simulink model "Boiler_System_Model"  (R2026a)
settings: Solver=ode15s  StopTime=1000
undefined symbols (not defined in the file): Flow_Min_LPM, P_Boost_W, P_Internal_W, Solar_Gain_Coeff, T_Ambient_C, T_Initial_C, T_Max_Cutoff_C, T_solar, T_standby, T_target_logic, T_Water_Inlet_C, UA_Losses, Water_Mass_kg
libraries: fl_lib x10, nesl_utility x7, simulink x3
settings Model: Creator=eladmual  LastModifiedBy=User
settings SolverCC: ZeroCrossAlgorithm=Adaptive
settings DebuggingCC: IgnoredZcDiagnostic=none
settings SimscapeCC: SimscapeNominalValues="[{\"value\":\"1\",\"unit\":\"A\"},{\"value\":\"1\",\"unit\":\"bar\"},{\"value\":\"1\",\"unit\":\"cm^2\"},{\"value\":\"1\",\"unit\":\"cm^3/s\"},{\"value\":\"1\",\"unit\":\"kJ/kg\"},{\"value\":\"1\",\"unit\":\"kW\"},{\"value\":\"1\",\"unit\":\"l\"},{\"value\":\"1\",\"unit\":\"N\"},{\"value\":\"1\",\"unit\":\"N*m\"},{\"value\":\"1\",\"unit\":\"V\"}]"  SimscapeLogType=none  SimscapeLogDataHistory=5000.0

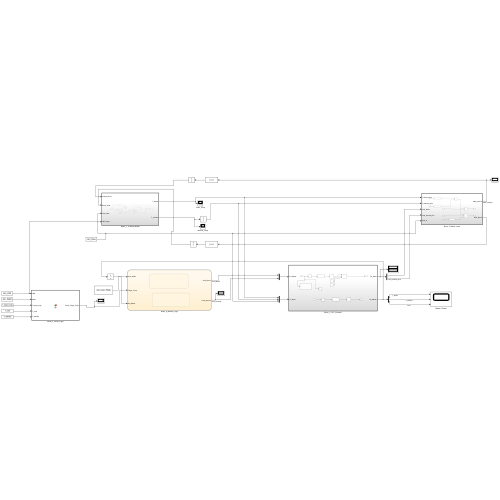
[thumbnail: Simulink's stored preview of the top-level diagram]
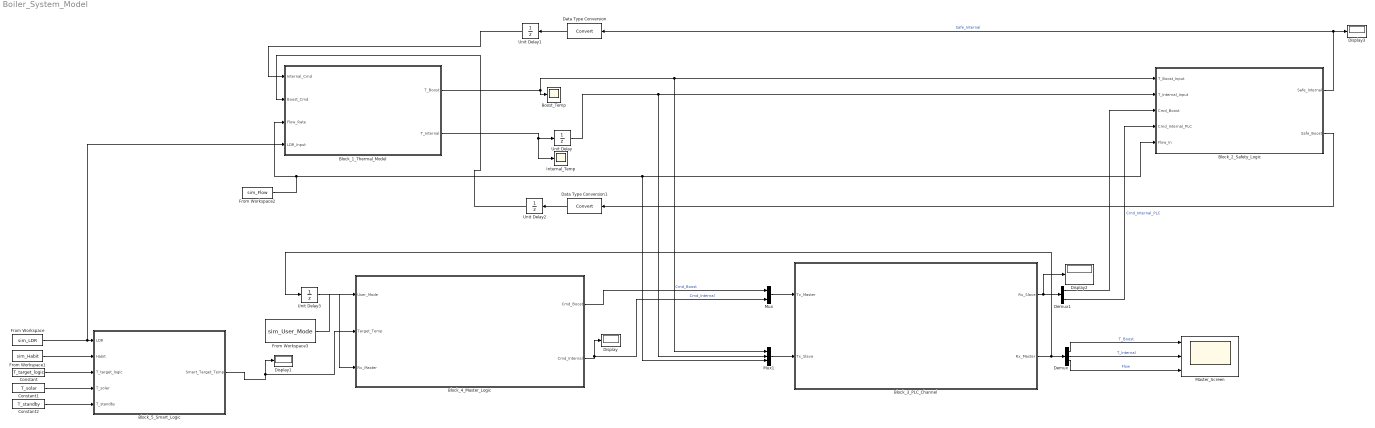
== system Boiler_System_Model ==
  Block_1_Thermal_Model : Subsystem  TreatAsAtomicUnit=on
  Block_2_Safety_Logic : Subsystem  TreatAsAtomicUnit=on
  Block_3_PLC_Channel : Subsystem  TreatAsAtomicUnit=on
  Block_4_Master_Logic : Stateflow chart  TreatAsAtomicUnit=on
  Block_5_Smart_Logic : MATLAB Function  TreatAsAtomicUnit=on
  Boost_Temp : Scope
      settings: ActiveDisplayYMinimum=8.9226285508408516  ActiveDisplayYMaximum=188.34662587796339
  Constant : Constant  Value=T_target_logic
  Constant1 : Constant  Value=T_solar
  Constant2 : Constant  Value=T_standby
  Data Type Conversion : DataTypeConversion  SaturateOnIntegerOverflow=off  RndMeth=Floor
  Data Type Conversion1 : DataTypeConversion  SaturateOnIntegerOverflow=off  RndMeth=Floor
  Demux : Demux  Outputs=3
  Demux1 : Demux  Outputs=2
  Display{,1..3} (4 alike) : Display
  From Workspace : FromWorkspace  VariableName=sim_LDR
  From Workspace1 : FromWorkspace  VariableName=sim_Habit
  From Workspace2 : FromWorkspace  VariableName=sim_Flow
  From Workspace3 : FromWorkspace  VariableName=sim_User_Mode
  Internal_Temp : Scope
      settings: ActiveDisplayYMinimum=25.95597381713398  ActiveDisplayYMaximum=34.896235645794405
  Master_Screen : Scope  NumInputPorts=3
      settings: ActiveDisplayYMinimum=0  ActiveDisplayYMaximum=70  DataLoggingVariableName=ScopeData2
  Mux : Mux  Inputs=2
  Mux1 : Mux  Inputs=3
  Unit Delay : UnitDelay  InitialCondition=20  SampleTime=-1
  Unit Delay1 : UnitDelay  InitialCondition=20  SampleTime=0.1
  Unit Delay2 : UnitDelay  InitialCondition=20  SampleTime=0.1
  Unit Delay3 : UnitDelay  SampleTime=-1
  wires:
  Block_1_Thermal_Model/2(T_Internal) -> Unit Delay/1, Internal_Temp/1
  From Workspace2/1 -> Mux1/3, Block_2_Safety_Logic/5(Flow_In), Block_1_Thermal_Model/3(Flow_Rate)
  Block_2_Safety_Logic/1(Safe_Internal) -> Data Type Conversion/1, Display3/1  "Safe_Internal"
  Block_2_Safety_Logic/2(Safe_Boost) -> Data Type Conversion1/1
  Data Type Conversion1/1 -> Unit Delay2/1
  Data Type Conversion/1 -> Unit Delay1/1
  Unit Delay/1 -> Mux1/2, Block_2_Safety_Logic/2(T_Internal_Input)
  Block_1_Thermal_Model/1(T_Boost) -> Boost_Temp/1, Mux1/1, Block_2_Safety_Logic/1(T_Boost_Input)
  Unit Delay1/1 -> Block_1_Thermal_Model/1(Internal_Cmd)
  Unit Delay2/1 -> Block_1_Thermal_Model/2(Boost_Cmd)
  Mux/1 -> Block_3_PLC_Channel/1(Tx_Master)
  Block_3_PLC_Channel/1(Rx_Slave) -> Display2/1, Demux1/1
  Mux1/1 -> Block_3_PLC_Channel/2(Tx_Slave)
  Demux/1 -> Master_Screen/1  "T_Boost"
  Demux/2 -> Master_Screen/2  "T_Internal"
  Demux/3 -> Master_Screen/3  "Flow"
  From Workspace3/1 -> Block_4_Master_Logic/1(User_Mode)
  Block_3_PLC_Channel/2(Rx_Master) -> Unit Delay3/1, Demux/1
  Block_4_Master_Logic/1(Cmd_Boost) -> Mux/1  "Cmd_Boost"
  Block_4_Master_Logic/2(Cmd_Internal) -> Display/1, Mux/2  "Cmd_Internal"
  Unit Delay3/1 -> Block_4_Master_Logic/3(Rx_Master)
  From Workspace/1 -> Block_5_Smart_Logic/1(LDR), Block_1_Thermal_Model/4(LDR_Input)
  From Workspace1/1 -> Block_5_Smart_Logic/2(Habit)
  Block_5_Smart_Logic/1(Smart_Target_Temp) -> Display1/1, Block_4_Master_Logic/2(Target_Temp)
  Demux1/1 -> Block_2_Safety_Logic/3(Cmd_Boost)
  Demux1/2 -> Block_2_Safety_Logic/4(Cmd_Internal_PLC)  "Cmd_Internal_PLC"
  Constant/1 -> Block_5_Smart_Logic/3(T_target_logic)
  Constant1/1 -> Block_5_Smart_Logic/4(T_solar)
  Constant2/1 -> Block_5_Smart_Logic/5(T_standby)

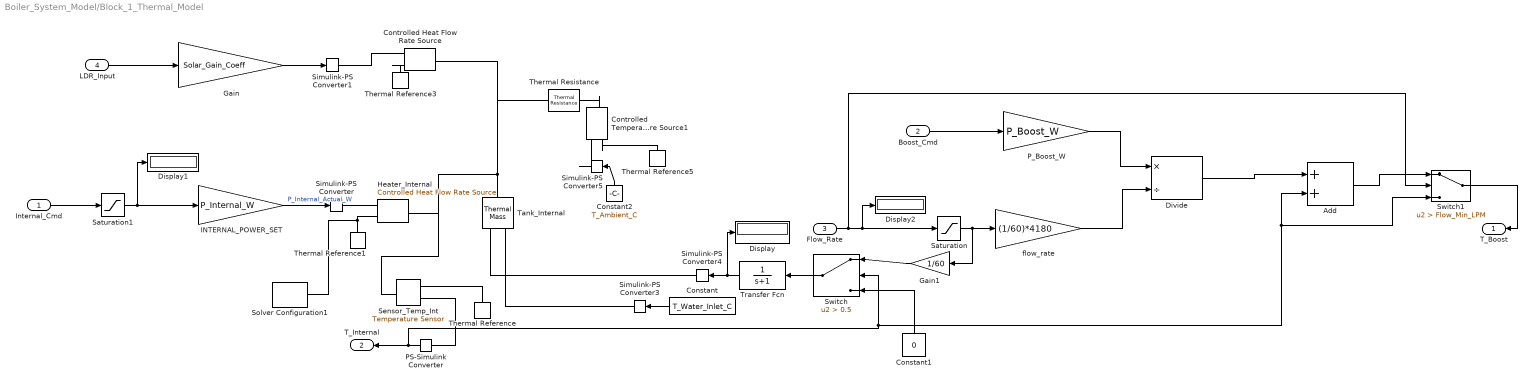
== system Boiler_System_Model/Block_1_Thermal_Model ==
  Internal_Cmd : Inport
  Boost_Cmd : Inport  Port=2
  Flow_Rate : Inport  Port=3
  LDR_Input : Inport  Port=4
  Add : Sum
  Constant : Constant  Value=T_Water_Inlet_C
  Constant1 : Constant  Value=0
  Constant2 : Constant  Value=T_Ambient_C
  Controlled Temperature Source1 : fl_lib/Thermal/Thermal Sources/Controlled Temperature Source
  Controlled Heat Flow Rate Source : fl_lib/Thermal/Thermal Sources/Controlled Heat Flow Rate Source
  Display : Display
  Display1 : Display
  Display2 : Display
  Divide : Product  Inputs=*/
  Gain : Gain  Gain=Solar_Gain_Coeff
  Gain1 : Gain  Gain=1/60
  Heater_Internal : fl_lib/Thermal/Thermal Sources/Controlled Heat Flow Rate Source
  INTERNAL_POWER_SET : Gain  Gain=P_Internal_W
  PS-Simulink Converter : nesl_utility/PS-Simulink Converter  PhysicalDomain=network_engine_domain  SubClassName=ps_output  LeftPortType=input  RightPortType=output  PseudoPeriodic=off  Frequencies=[]  VectorFormat=inherit  Unit=degC  AffineConversion=on
  P_Boost_W : Gain  Gain=P_Boost_W
  Saturation : Saturate  UpperLimit=inf  LowerLimit=0.001
  Saturation1 : Saturate  UpperLimit=1  LowerLimit=0
  Sensor_Temp_Int : fl_lib/Thermal/Thermal Sensors/Temperature Sensor  temperature_measure=foundation.enum.MeasurementReference.difference
  Simulink-PS Converter : nesl_utility/Simulink-PS Converter  PhysicalDomain=network_engine_domain  SubClassName=ps_input  LeftPortType=input  RightPortType=output  PseudoPeriodic=off  Frequencies=[]  NoiseDistribution=none  NoiseParameters=[]  Unit=W  AffineConversion=on  FilteringAndDerivatives=provide  SimscapeFilterOrder=1  InputFilterTimeConstant=0.001  UdotUserProvided=0
  Simulink-PS Converter1 : nesl_utility/Simulink-PS Converter  PhysicalDomain=network_engine_domain  SubClassName=ps_input  LeftPortType=input  RightPortType=output  PseudoPeriodic=off  Frequencies=[]  NoiseDistribution=none  NoiseParameters=[]  Unit=1  AffineConversion=off  FilteringAndDerivatives=provide  SimscapeFilterOrder=1  InputFilterTimeConstant=0.001  UdotUserProvided=0
  Simulink-PS Converter3 : nesl_utility/Simulink-PS Converter  PhysicalDomain=network_engine_domain  SubClassName=ps_input  LeftPortType=input  RightPortType=output  PseudoPeriodic=off  Frequencies=[]  NoiseDistribution=none  NoiseParameters=[]  Unit=1  AffineConversion=off  FilteringAndDerivatives=provide  SimscapeFilterOrder=1  InputFilterTimeConstant=0.001  UdotUserProvided=0
  Simulink-PS Converter4 : nesl_utility/Simulink-PS Converter  PhysicalDomain=network_engine_domain  SubClassName=ps_input  LeftPortType=input  RightPortType=output  PseudoPeriodic=off  Frequencies=[]  NoiseDistribution=none  NoiseParameters=[]  Unit=1  AffineConversion=off  FilteringAndDerivatives=provide  SimscapeFilterOrder=1  InputFilterTimeConstant=0.001  UdotUserProvided=0
  Simulink-PS Converter5 : nesl_utility/Simulink-PS Converter  PhysicalDomain=network_engine_domain  SubClassName=ps_input  LeftPortType=input  RightPortType=output  PseudoPeriodic=off  Frequencies=[]  NoiseDistribution=none  NoiseParameters=[]  Unit=degC  AffineConversion=on  FilteringAndDerivatives=provide  SimscapeFilterOrder=1  InputFilterTimeConstant=0.001  UdotUserProvided=0
  Solver Configuration1 : nesl_utility/Solver Configuration  PhysicalDomain=network_engine_domain  SubClassName=solver  LeftPortType=input  RightPortType=generic  Tones=[]  Harmonics=[]  SimulateNoise=off  Profile=off  UseLocalSampling=off  EnableSwitchedLinearOptims=on  FrequencyDomain=off  UseCCode=off  RelTol=0.001  AbsTol=0.001  MinStep=1e-09  ToWorkspace=off  RevertToSquareIcSolve=off  NumHomotopyIterations=100  PhasorMode=off  PhasorModeNumHarmonics=1  ConsistencySolver=NEWTON_XTOL_AFTER_FTOL  CanonicalOrdering=UNORDERED  OptimizeIntermediates=UNOPTIMIZED  IndexReductionMethod=DerivativeReplacement  DoDC=off  ResidualTolerance=1e-09  ConsistencyTolSource=GLOBAL  ConsistencyAbsTol=0.001  ConsistencyRelTol=0.001  ConsistencyTolFactor=0.001  UseLocalSolver=off  LocalSolverChoice=NE_BACKWARD_EULER_ADVANCER  ResolveIndetEquations=on  FunctionEvalNumThread=1  LocalSolverSampleTime=0.001  DoFixedCost=off  MaxNonlinIter=3  MaxModeIter=2  ComputeImpulses=off  ImpulseIterations=2  LinearAlgebra=auto  LinearAlgebraNumThread=0  EquationFormulation=NE_TIME_EF  DelaysMemoryBudget=1024  AutomaticFiltering=on  FilteringTimeConstant=0.001  PartitionStorageMethod=AS_NEEDED  PartitionMemoryBudget=1024  PartitionMethod=ROBUST  MultibodyUseLocalSolver=off  MultibodyLocalSolverChoice=ODE1  MultibodyLocalSolverSampleTime=0.001
  Switch : Switch  Criteria=u2 > Threshold  Threshold=0.5  ZeroCross=off  SaturateOnIntegerOverflow=off  InputSameDT=off
  Switch1 : Switch  Criteria=u2 > Threshold  Threshold=Flow_Min_LPM  SaturateOnIntegerOverflow=off  InputSameDT=off
  Tank_Internal : fl_lib/Thermal/Thermal Elements/Thermal Mass  mass_type=foundation.enum.constant_variable.variable  mass=Water_Mass_kg kg  sp_heat=4184 J/(K*kg)  mass_min=1 kg  num_ports=foundation.enum.numPorts2.one  m_specify=on  m_priority=High  m=Water_Mass_kg kg  m_nominal_specify=off  m_nominal_value=1  m_nominal_unit=kg  T_specify=on  T_priority=High  T=T_Initial_C degC  T_nominal_specify=off  T_nominal_value=1  T_nominal_unit=K  Q_specify=off  Q_priority=None  Q=0 W  Q_nominal_specify=off  Q_nominal_value=1  Q_nominal_unit=W
  Thermal Reference{,1,3,5} (4 alike) : fl_lib/Thermal/Thermal Elements/Thermal Reference
  Thermal Resistance : fl_lib/Thermal/Thermal Elements/Thermal Resistance  resistance=1/UA_Losses K/W  T_specify=off  T_priority=None  T=0 K  T_nominal_specify=off  T_nominal_value=1  T_nominal_unit=K  Q_specify=off  Q_priority=None  Q=0 W  Q_nominal_specify=off  Q_nominal_value=1  Q_nominal_unit=W
  Transfer Fcn : TransferFcn  Denominator=[1 1]
  flow_rate : Gain  Gain=(1/60)*4180
  T_Boost : Outport  Unit=degC
  T_Internal : Outport  Port=2  Unit=°C
  wires:
  Boost_Cmd/1 -> P_Boost_W/1
  INTERNAL_POWER_SET/1 -> Simulink-PS Converter/1  "P_Internal_Actual_W"
  P_Boost_W/1 -> Divide/1
  flow_rate/1 -> Divide/2
  PS-Simulink Converter/1 -> Switch/2, Switch1/3, Add/2, T_Internal/1
  Divide/1 -> Add/1
  LDR_Input/1 -> Gain/1
  Flow_Rate/1 -> Switch1/2, Display2/1, Saturation/1
  Saturation/1 -> Gain1/1, flow_rate/1
  Gain/1 -> Simulink-PS Converter1/1
  Constant/1 -> Simulink-PS Converter3/1
  Gain1/1 -> Switch/1
  Constant1/1 -> Switch/3
  Switch/1 -> Transfer Fcn/1
  Transfer Fcn/1 -> Display/1, Simulink-PS Converter4/1
  Add/1 -> Switch1/1
  Constant2/1 -> Simulink-PS Converter5/1
  Internal_Cmd/1 -> Saturation1/1
  Saturation1/1 -> INTERNAL_POWER_SET/1, Display1/1
  Switch1/1 -> T_Boost/1
  connections:
  Sensor_Temp_Int/LConn1 -- Heater_Internal/LConn1 -- Thermal Resistance/LConn1 -- Controlled Heat Flow Rate Source/LConn1 -- Tank_Internal/LConn1
  Simulink-PS Converter/RConn1 -- Heater_Internal/RConn1
  PS-Simulink Converter/LConn1 -- Sensor_Temp_Int/RConn2
  Heater_Internal/RConn2 -- Solver Configuration1/RConn1 -- Thermal Reference1/LConn1
  Sensor_Temp_Int/RConn1 -- Thermal Reference/LConn1
  Controlled Heat Flow Rate Source/RConn1 -- Simulink-PS Converter1/RConn1
  Controlled Heat Flow Rate Source/RConn2 -- Thermal Reference3/LConn1
  Tank_Internal/RConn2 -- Simulink-PS Converter3/RConn1
  Tank_Internal/RConn1 -- Simulink-PS Converter4/RConn1
  Controlled Temperature Source1/LConn1 -- Thermal Resistance/RConn1
  Simulink-PS Converter5/RConn1 -- Controlled Temperature Source1/RConn1
  Controlled Temperature Source1/RConn2 -- Thermal Reference5/LConn1

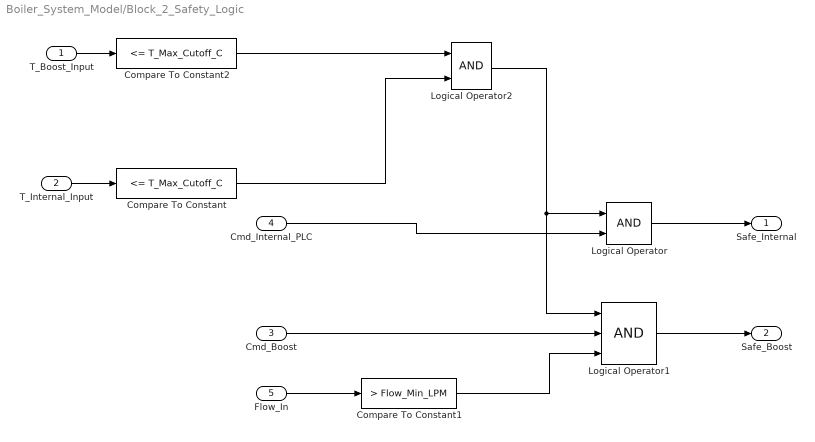
== system Boiler_System_Model/Block_2_Safety_Logic ==
  T_Boost_Input : Inport
  T_Internal_Input : Inport  Port=2  Unit=°C
  Cmd_Boost : Inport  Port=3
  Cmd_Internal_PLC : Inport  Port=4
  Flow_In : Inport  Port=5
  Compare To Constant : simulink/Logic and Bit Operations/Compare To Constant  relop=<=  const=T_Max_Cutoff_C  OutDataTypeStr=boolean
  Compare To Constant1 : simulink/Logic and Bit Operations/Compare To Constant  relop=>  const=Flow_Min_LPM  OutDataTypeStr=boolean
  Compare To Constant2 : simulink/Logic and Bit Operations/Compare To Constant  relop=<=  const=T_Max_Cutoff_C  OutDataTypeStr=boolean
  Logical Operator : Logic  AllPortsSameDT=off  OutDataTypeStr=boolean
  Logical Operator1 : Logic  Inputs=3  AllPortsSameDT=off  OutDataTypeStr=boolean
  Logical Operator2 : Logic  AllPortsSameDT=off  OutDataTypeStr=boolean
  Safe_Internal : Outport
  Safe_Boost : Outport  Port=2
  wires:
  Cmd_Internal_PLC/1 -> Logical Operator/2
  Logical Operator/1 -> Safe_Internal/1
  T_Internal_Input/1 -> Compare To Constant/1
  Compare To Constant/1 -> Logical Operator2/2
  Flow_In/1 -> Compare To Constant1/1
  Compare To Constant1/1 -> Logical Operator1/3
  Logical Operator1/1 -> Safe_Boost/1
  T_Boost_Input/1 -> Compare To Constant2/1
  Compare To Constant2/1 -> Logical Operator2/1
  Cmd_Boost/1 -> Logical Operator1/2
  Logical Operator2/1 -> Logical Operator1/1, Logical Operator/1

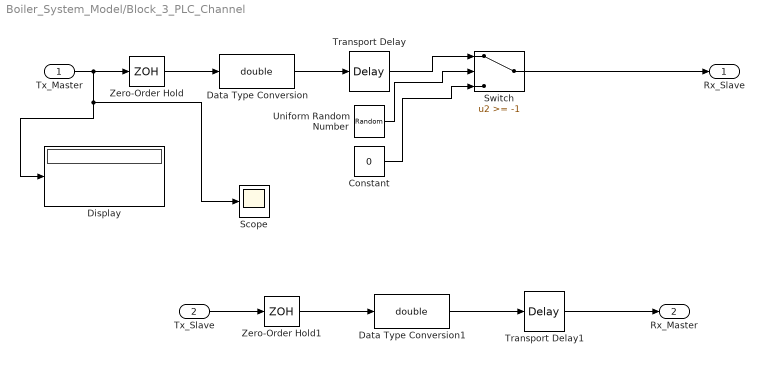
== system Boiler_System_Model/Block_3_PLC_Channel ==
  Tx_Master : Inport
  Tx_Slave : Inport  Port=2
  Constant : Constant  Value=0
  Data Type Conversion : DataTypeConversion  OutDataTypeStr=double  SaturateOnIntegerOverflow=off  RndMeth=Floor
  Data Type Conversion1 : DataTypeConversion  OutDataTypeStr=double  SaturateOnIntegerOverflow=off  RndMeth=Floor
  Display : Display
  Scope : Scope
      settings: ActiveDisplayYMinimum=-1  ActiveDisplayYMaximum=1  DataLoggingVariableName=ScopeData3
  Switch : Switch  Threshold=-1  SaturateOnIntegerOverflow=off  InputSameDT=off
  Transport Delay : TransportDelay  DelayTime=0.2  BufferSize=8192
  Transport Delay1 : TransportDelay  DelayTime=0.2  BufferSize=8192
  Uniform Random Number : UniformRandomNumber  SampleTime=0.1
  Zero-Order Hold : ZeroOrderHold  SampleTime=0.01
  Zero-Order Hold1 : ZeroOrderHold  SampleTime=0.01
  Rx_Slave : Outport
  Rx_Master : Outport  Port=2
  wires:
  Tx_Master/1 -> Zero-Order Hold/1, Scope/1, Display/1
  Zero-Order Hold/1 -> Data Type Conversion/1
  Zero-Order Hold1/1 -> Data Type Conversion1/1
  Tx_Slave/1 -> Zero-Order Hold1/1
  Transport Delay/1 -> Switch/1
  Uniform Random Number/1 -> Switch/2
  Constant/1 -> Switch/3
  Data Type Conversion/1 -> Transport Delay/1
  Switch/1 -> Rx_Slave/1
  Data Type Conversion1/1 -> Transport Delay1/1
  Transport Delay1/1 -> Rx_Master/1

== matlab function Boiler_System_Model/Block_5_Smart_Logic ==
  data: LDR input; Smart_Target_Temp output; Habit input; T_target_logic input; T_solar input; T_standby input
function Smart_Target_Temp = fcn(LDR, Habit, T_target_logic, T_solar, T_standby)
    % This function determines the dynamic temperature setpoint
    % based on user habits and environmental conditions (Solar Bypass).
    
    if (Habit > 0.5)
        % PRIORITY 1: Active user demand (Shower/Habit)
        % Set to main comfort target (e.g., 40C)
        Smart_Target_Temp = T_target_logic;
        
    elseif (LDR > 70)
        % PRIORITY 2: High Solar Radiation Detected
        % Predictive Solar Bypass: Lower the electric target (e.g., 20C)
        % to allow natural solar gain without triggering electric heaters.
        Smart_Target_Temp = T_solar;
        
    else
        % PRIORITY 3: Idle / Standby Mode
        % Maintain standard standby temperature
        Smart_Target_Temp = T_standby;
    end
end

== stateflow chart Boiler_System_Model/Block_4_Master_Logic ==
  state Control_Task [parallel]
    during:
    % 1. Boost Logic: Active only when flow is detected and immediate hot water is needed
    Cmd_Boost = (User_Mode == 1) && (Rx_Master(3) > 1) && (Rx_Master(2) < 40);
    % 2. Internal Tank Logic: Uses smart target from Block 5 with Load Shedding interlock
    % Internal heater is automatically disabled whenever Boost is active to prevent overcurrent
    Cmd_Internal = (Rx_Master(2) < Target_Temp) && ~Cmd_Boost;
    settings: executionOrder=1
  state Safety_Task [parallel]
    during:
    % Emergency software shutdown if tank temperature exceeds 95 degrees Celsius
    if Rx_Master(2) > 90
    Cmd_Internal = false; % Forcefully disable internal heater
    Cmd_Boost = false;    % Forcefully disable boost heater
    end
    settings: executionOrder=2
  data: User_Mode input; Target_Temp input; Rx_Master input; Cmd_Boost output; Cmd_Internal output
